simulink model "planta_2_Ku"  (R2018b)
settings: Solver=VariableStepAuto  StartTime=0.0  StopTime=10.0  RelTol=1e-3
settings Model: Creator=fpassold  LastModifiedBy=fpassold

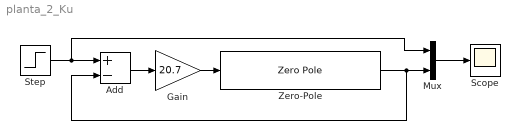
== system planta_2_Ku ==
  Add : Sum  Inputs=+-
  Gain : Gain  Gain=20.7
  Mux : Mux  Inputs=2
  Scope : Scope
  Step : Step  SampleTime=0
  Zero-Pole : ZeroPole  Zeros=[ ]  Poles=[-1 -4 -12]  Gain=[48]
  wires:
  Step/1 -> Mux/1, Add/1
  Add/1 -> Gain/1
  Gain/1 -> Zero-Pole/1
  Mux/1 -> Scope/1
  Zero-Pole/1 -> Mux/2, Add/2
